simulink model "Grue_NL_corrNL"  (R2018b)
settings: Solver=ode1  StartTime=0.0  StopTime=dt  FixedStep=1e-2  RelTol=1e-3  EnableMultiTasking=on
values from neighbouring files (symbols this model uses):
  a = (Rini-zh)/(Dini-xh)^2    [Ini_Grue.m]
  b = 0.4    [Ini_Grue.m]
  C0 = m*g*b    (= 2000)    [Ini_Grue.m]
  Cd = 20    [Ini_Grue.m]
  coeff_phi = [6/Deltat^5 -15/Deltat^4 10/Deltat^3 0 0 0]    [Ini_Grue.m]
  coeff_phi2 = [-20/Deltat^7 70/Deltat^6 -84/Deltat^5 35/Deltat^4 0 0 0 0]    [Ini_Grue.m]
  Cr = 20    [Ini_Grue.m]    (also in plot_things.m = Cr*kc)
  Dfin = 20    [Ini_Grue.m]
  Dini = 0    [Ini_Grue.m]
  ed = omega0/100    [Ini_Grue.m]    (also in plot_things.m = omega0/e)
  er = ed    [Ini_Grue.m]    (also in plot_things.m = omega0/e)
  g = 10    [Ini_Grue.m]
  J = 50    [Ini_Grue.m]
  m = 500    [Ini_Grue.m]    (also in plot_things.m)
  Mc = 5000    [Ini_Grue.m]
  R = 15    [Ini_Grue.m]
  Rfin = 15    [Ini_Grue.m]
  Rini = 15    [Ini_Grue.m]
  xh = (Dini+sqrt((Rini-zh)/(Rfin-zh))*Dfin)/(1+sqrt((Rini-zh)/(Rfin-zh)))    [Ini_Grue.m]
  zh = 1    [Ini_Grue.m]
settings Model: Creator=abbasturki  LastModifiedBy=pac
settings DataIOCC: LimitDataPoints=on  SaveFormat=Array  SignalLoggingSaveFormat=ModelDataLogs
settings OptimizationCC: ExpressionDepthLimit=2147483647  LifeSpan=inf
settings DebuggingCC: UnderspecifiedInitializationDetection=Classic  MergeDetectMultiDrivingBlocksExec=none  SolverPrmCheckMsg=warning  FcnCallInpInsideContextMsg=warning  StateNameClashWarn=warning  SFUnexpectedBacktrackingDiag=warning  SFNoUnconditionalDefaultTransitionDiag=warning  SFExecutionAtInitializationDiag=none
settings HardwareCC: ProdBitPerPointer=32  ProdBitPerSizeT=32  ProdBitPerPtrDiffT=32  ProdLargestAtomicFloat=None  ProdIntDivRoundTo=Undefined  ProdEndianess=Unspecified  ProdWordSize=32  ProdHWDeviceType=32-bit Generic
settings ModelReferenceCC: PropagateSignalLabelsOutOfModel=off
settings SFSimCC: SimUseLocalCustomCode=off
settings RTWCC: RTWUseLocalCustomCode=off
settings CodeAppCC: StateflowObjectComments=on
settings GRTTargetCC: TargetLangStandard=C89/C90 (ANSI)  GeneratePreprocessorConditionals=Disable all  CombineOutputUpdateFcns=off  GRTInterface=on
settings ConfigComp: CovMetricSettings=dw  CovHtmlReporting=on  CovSaveCumulativeToWorkspaceVar=on  CovSaveSingleToWorkspaceVar=on  CovExternalEMLEnable=off

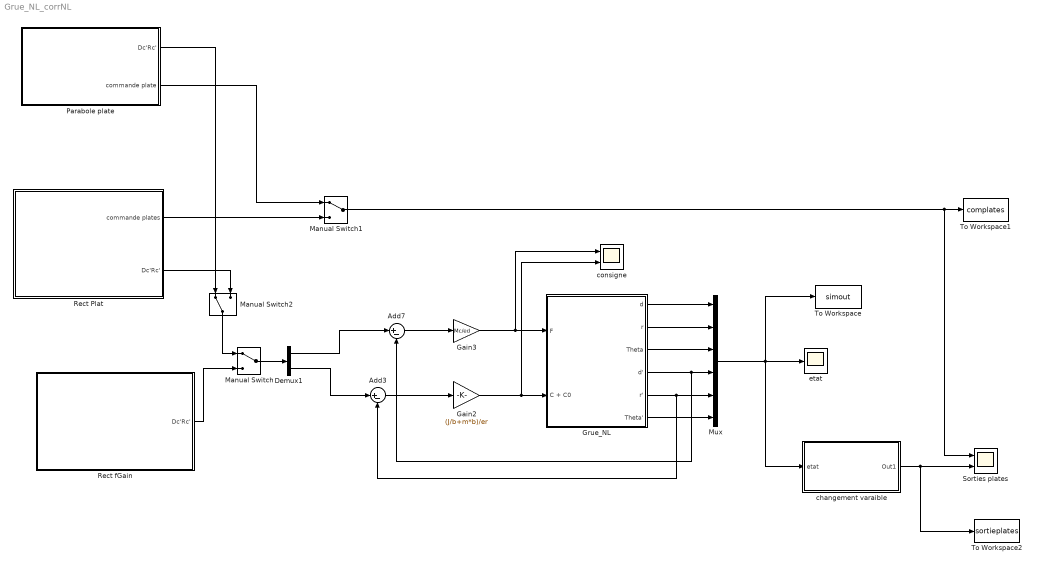
== system Grue_NL_corrNL ==
  Add3 : Sum  Inputs=|+-
  Add7 : Sum  Inputs=|+-
  Demux1 : Demux  Outputs=2
  Gain2 : Gain  Gain=(J/b+m*b)/er
  Gain3 : Gain  Gain=Mc/ed
  Grue_NL : Subsystem
  Manual Switch : ManualSwitch
  Manual Switch1 : ManualSwitch
  Manual Switch2 : ManualSwitch
  Mux : Mux  Inputs=6
  Parabole plate : Subsystem
  Rect Plat : Subsystem
  "Rect fGain " : Subsystem
  Sorties plates : Scope  NumInputPorts=2
  To Workspace : ToWorkspace  VariableName=simout  SaveFormat=Timeseries  SampleTime=-1
  To Workspace1 : ToWorkspace  VariableName=complates  SaveFormat=Timeseries  SampleTime=-1
  To Workspace2 : ToWorkspace  VariableName=sortieplates  SaveFormat=Timeseries  SampleTime=-1
  changement varaible : Subsystem
  consigne : Scope  NumInputPorts=2
  etat : Scope
  wires:
  Grue_NL/1(d) -> Mux/1
  Grue_NL/2(r) -> Mux/2
  Grue_NL/3(Theta) -> Mux/3
  Grue_NL/6(Theta') -> Mux/6
  Mux/1 -> changement varaible/1(etat), etat/1, To Workspace/1
  Gain3/1 -> consigne/1, Grue_NL/1(F)
  Gain2/1 -> consigne/2, Grue_NL/2(C + C0)
  Add7/1 -> Gain3/1
  Grue_NL/5(r') -> Add3/2, Mux/5
  Grue_NL/4(d') -> Add7/2, Mux/4
  Add3/1 -> Gain2/1
  Manual Switch/1 -> Demux1/1
  "Rect fGain "/1(Dc'Rc') -> Manual Switch/2
  Demux1/1 -> Add7/1
  Demux1/2 -> Add3/1
  changement varaible/1(Out1) -> To Workspace2/1, Sorties plates/2
  Parabole plate/2(commande plate) -> Manual Switch1/1
  Rect Plat/1(commande plates) -> Manual Switch1/2
  Manual Switch1/1 -> Sorties plates/1, To Workspace1/1
  Manual Switch2/1 -> Manual Switch/1
  Rect Plat/2(Dc'Rc') -> Manual Switch2/2
  Parabole plate/1(Dc'Rc') -> Manual Switch2/1

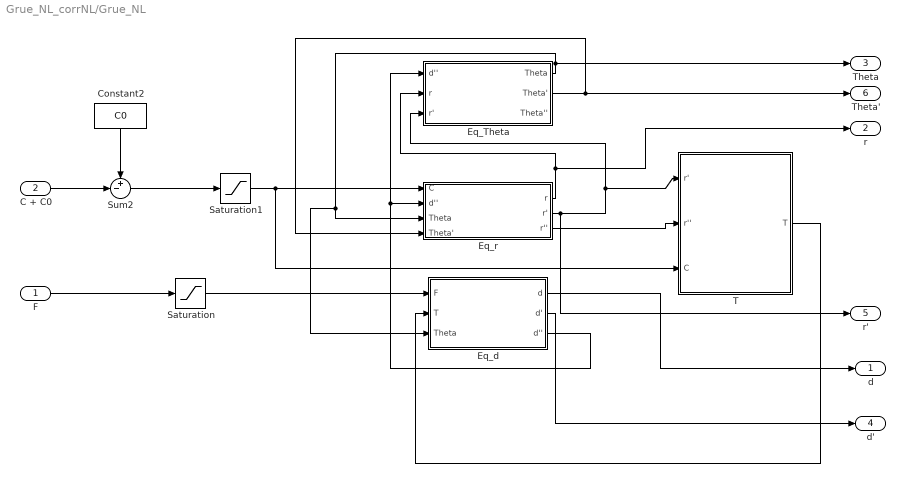
== system Grue_NL_corrNL/Grue_NL ==
  F : Inport
  C + C0 : Inport  Port=2
  Constant2 : Constant  Value=C0
  Eq_Theta : Subsystem
  Eq_d : Subsystem
  Eq_r : Subsystem
  Saturation : Saturate  UpperLimit=1e4  LowerLimit=-1e4
  Saturation1 : Saturate  UpperLimit=3e3  LowerLimit=-3e3
  Sum2 : Sum  Inputs=+-|
  T : Subsystem
  d : Outport
  r : Outport  Port=2
  Theta : Outport  Port=3
  d' : Outport  Port=4
  r' : Outport  Port=5
  Theta' : Outport  Port=6
  wires:
  Eq_r/2(r') -> Eq_Theta/3(r'), T/1(r'), r'/1
  Eq_r/1(r) -> Eq_Theta/2(r), r/1
  Eq_d/3(d'') -> Eq_Theta/1(d''), Eq_r/2(d'')
  Eq_d/2(d') -> d'/1
  Eq_Theta/1(Theta) -> Eq_d/3(Theta), Eq_r/3(Theta), Theta/1
  Eq_Theta/2(Theta') -> Eq_r/4(Theta'), Theta'/1
  Eq_r/3(r'') -> T/2(r'')
  F/1 -> Saturation/1
  T/1(T) -> Eq_d/2(T)
  Eq_d/1(d) -> d/1
  Saturation/1 -> Eq_d/1(F)
  Saturation1/1 -> Eq_r/1(C), T/3(C)
  Constant2/1 -> Sum2/1
  Sum2/1 -> Saturation1/1
  C + C0/1 -> Sum2/2

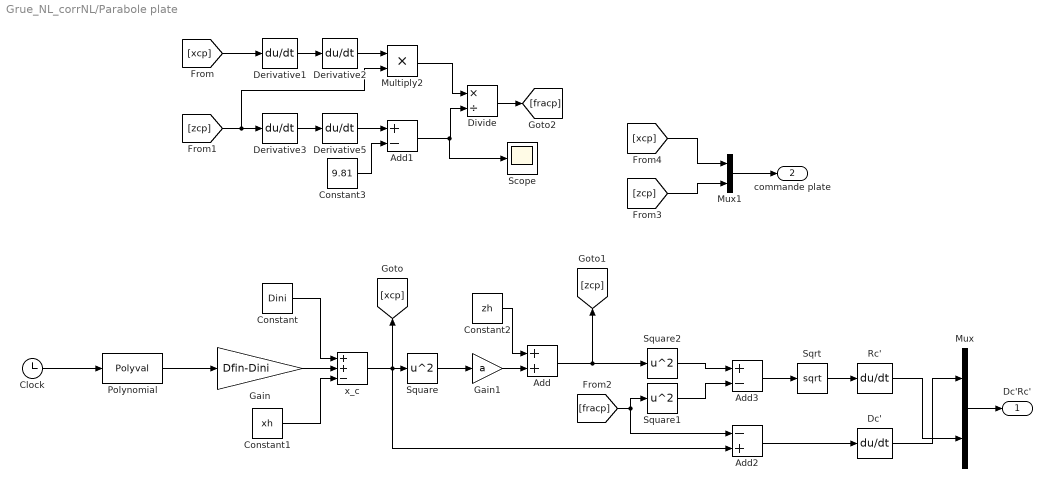
== system Grue_NL_corrNL/Parabole plate ==
  Add : Sum
  Add1 : Sum  Inputs=+-
  Add2 : Sum  Inputs=-+
  Add3 : Sum  Inputs=+-
  Clock : Clock
  Constant : Constant  Value=Dini
  Constant1 : Constant  Value=xh
  Constant2 : Constant  Value=zh
  Constant3 : Constant  Value=9.81
  Dc' : Derivative
  Derivative{1..3,5} (4 alike) : Derivative
  Divide : Product  Inputs=*/
  Gain : Gain  Gain=Dfin-Dini
  Gain1 : Gain  Gain=a
  Multiply2 : Product
  Mux : Mux  Inputs=2
  Mux1 : Mux  Inputs=2
  Polynomial : Polyval  Coefs=coeff_phi2
  Rc' : Derivative
  Scope : Scope
  Sqrt : Sqrt  SaturateOnIntegerOverflow=on
  Square : Math  Operator=square  SaturateOnIntegerOverflow=on
  Square1 : Math  Operator=square  SaturateOnIntegerOverflow=on
  Square2 : Math  Operator=square  SaturateOnIntegerOverflow=on
  x_c : Sum  Inputs=++-
  Dc'Rc' : Outport
  commande plate : Outport  Port=2
  wires:
  Constant/1 -> x_c/1
  Polynomial/1 -> Gain/1
  Square/1 -> Gain1/1
  Gain1/1 -> Add/2
  Gain/1 -> x_c/2
  Constant1/1 -> x_c/3
  Constant2/1 -> Add/1
  Clock/1 -> Polynomial/1
  Derivative2/1 -> Multiply2/1
  Divide/1 -> [fracp]
  Derivative3/1 -> Derivative5/1
  Derivative1/1 -> Derivative2/1
  [zcp] -> Multiply2/2, Derivative3/1
  Multiply2/1 -> Divide/1
  Add1/1 -> Scope/1, Divide/2
  Constant3/1 -> Add1/2
  Derivative5/1 -> Add1/1
  [xcp] -> Derivative1/1
  x_c/1 -> Add2/2, [xcp], Square/1
  [fracp] -> Add2/1, Square1/1
  Rc'/1 -> Mux/2
  Add2/1 -> Dc'/1
  Mux/1 -> Dc'Rc'/1
  Dc'/1 -> Mux/1
  Sqrt/1 -> Rc'/1
  Add/1 -> [zcp], Square2/1
  Square2/1 -> Add3/1
  Square1/1 -> Add3/2
  Add3/1 -> Sqrt/1
  Mux1/1 -> commande plate/1
  [xcp] -> Mux1/1
  [zcp] -> Mux1/2

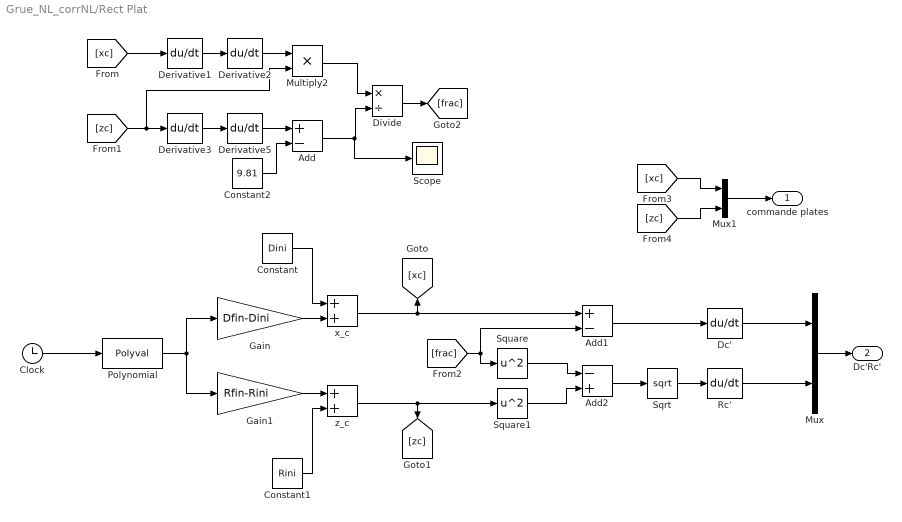
== system Grue_NL_corrNL/Rect Plat ==
  Add : Sum  Inputs=+-
  Add1 : Sum  Inputs=+-
  Add2 : Sum  Inputs=-+
  Clock : Clock
  Constant : Constant  Value=Dini
  Constant1 : Constant  Value=Rini
  Constant2 : Constant  Value=9.81
  Dc' : Derivative
  Derivative{1..3,5} (4 alike) : Derivative
  Divide : Product  Inputs=*/
  Gain : Gain  Gain=Dfin-Dini
  Gain1 : Gain  Gain=Rfin-Rini
  Multiply2 : Product
  Mux : Mux  Inputs=2
  Mux1 : Mux  Inputs=2
  Polynomial : Polyval  Coefs=coeff_phi2
  Rc' : Derivative
  Scope : Scope
  Sqrt : Sqrt  SaturateOnIntegerOverflow=on
  Square : Math  Operator=square  SaturateOnIntegerOverflow=on
  Square1 : Math  Operator=square  SaturateOnIntegerOverflow=on
  x_c : Sum
  z_c : Sum
  commande plates : Outport
  Dc'Rc' : Outport  Port=2
  wires:
  Gain1/1 -> z_c/1
  Square/1 -> Add2/1
  Derivative2/1 -> Multiply2/1
  Sqrt/1 -> Rc'/1
  Rc'/1 -> Mux/2
  Add2/1 -> Sqrt/1
  Add/1 -> Scope/1, Divide/2
  [zc] -> Multiply2/2, Derivative3/1
  Add1/1 -> Dc'/1
  z_c/1 -> Square1/1, [zc]
  Clock/1 -> Polynomial/1
  Polynomial/1 -> Gain/1, Gain1/1
  Multiply2/1 -> Divide/1
  Dc'/1 -> Mux/1
  Derivative3/1 -> Derivative5/1
  Derivative1/1 -> Derivative2/1
  Constant2/1 -> Add/2
  [xc] -> Derivative1/1
  Gain/1 -> x_c/2
  x_c/1 -> Add1/1, [xc]
  Constant1/1 -> z_c/2
  Constant/1 -> x_c/1
  Derivative5/1 -> Add/1
  Square1/1 -> Add2/2
  Divide/1 -> [frac]
  [frac] -> Add1/2, Square/1
  Mux/1 -> Dc'Rc'/1
  [xc] -> Mux1/1
  [zc] -> Mux1/2
  Mux1/1 -> commande plates/1

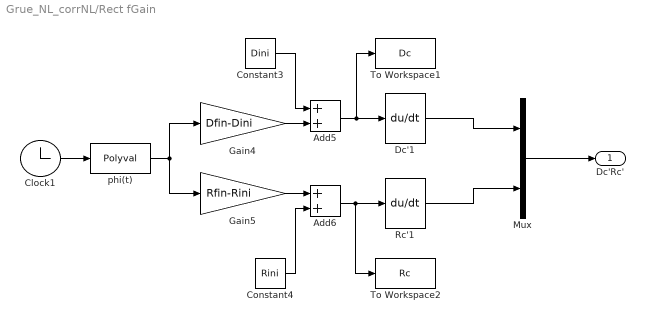
== system Grue_NL_corrNL/Rect fGain  ==
  Add5 : Sum
  Add6 : Sum
  Clock1 : Clock
  Constant3 : Constant  Value=Dini
  Constant4 : Constant  Value=Rini
  Dc'1 : Derivative
  Gain4 : Gain  Gain=Dfin-Dini
  Gain5 : Gain  Gain=Rfin-Rini
  Mux : Mux  Inputs=2
  Rc'1 : Derivative
  To Workspace1 : ToWorkspace  VariableName=Dc  SaveFormat=Timeseries  SampleTime=-1
  To Workspace2 : ToWorkspace  VariableName=Rc  SaveFormat=Timeseries  SampleTime=-1
  phi(t) : Polyval  Coefs=coeff_phi
  Dc'Rc' : Outport
  wires:
  Constant4/1 -> Add6/2
  Gain5/1 -> Add6/1
  Clock1/1 -> phi(t)/1
  Add5/1 -> To Workspace1/1, Dc'1/1
  Constant3/1 -> Add5/1
  Add6/1 -> To Workspace2/1, Rc'1/1
  phi(t)/1 -> Gain4/1, Gain5/1
  Gain4/1 -> Add5/2
  Rc'1/1 -> Mux/2
  Mux/1 -> Dc'Rc'/1
  Dc'1/1 -> Mux/1

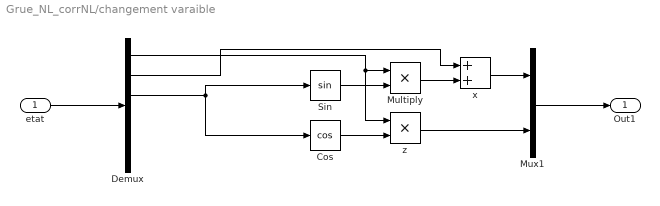
== system Grue_NL_corrNL/changement varaible ==
  etat : Inport
  Cos : Trigonometry  Operator=cos
  Demux : Demux  Outputs=6
  Multiply : Product
  Mux1 : Mux  Inputs=2
  Sin : Trigonometry
  x : Sum
  z : Product
  Out1 : Outport
  wires:
  Cos/1 -> z/2
  Multiply/1 -> x/2
  Sin/1 -> Multiply/2
  Demux/3 -> Cos/1, Sin/1
  z/1 -> Mux1/2
  Mux1/1 -> Out1/1
  etat/1 -> Demux/1
  Demux/1 -> z/1, Multiply/1
  x/1 -> Mux1/1
  Demux/2 -> x/1

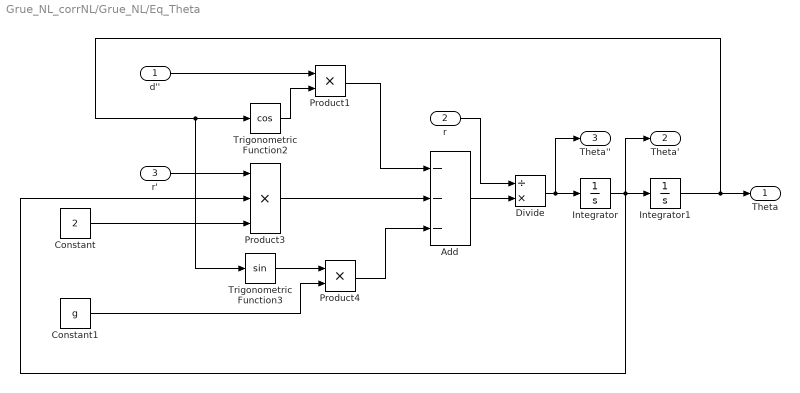
== system Grue_NL_corrNL/Grue_NL/Eq_Theta ==
  d'' : Inport
  r : Inport  Port=2
  r' : Inport  Port=3
  Add : Sum  Inputs=---
  Constant : Constant  Value=2
  Constant1 : Constant  Value=g
  Divide : Product  Inputs=/*
  Integrator : Integrator
  Integrator1 : Integrator
  Product1 : Product  RndMeth=Zero
  Product3 : Product  Inputs=3  RndMeth=Zero
  Product4 : Product  RndMeth=Zero
  Trigonometric Function2 : Trigonometry  Operator=cos
  Trigonometric Function3 : Trigonometry
  Theta : Outport
  Theta' : Outport  Port=2
  Theta'' : Outport  Port=3
  wires:
  d''/1 -> Product1/1
  Trigonometric Function2/1 -> Product1/2
  r'/1 -> Product3/1
  Constant/1 -> Product3/3
  Trigonometric Function3/1 -> Product4/1
  Constant1/1 -> Product4/2
  Product1/1 -> Add/1
  Product3/1 -> Add/2
  Product4/1 -> Add/3
  r/1 -> Divide/1
  Add/1 -> Divide/2
  Divide/1 -> Integrator/1, Theta''/1
  Integrator/1 -> Integrator1/1, Product3/2, Theta'/1
  Integrator1/1 -> Theta/1, Trigonometric Function2/1, Trigonometric Function3/1

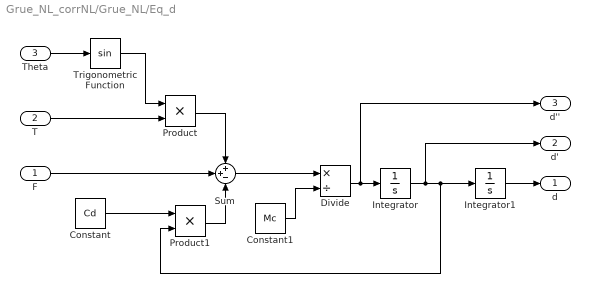
== system Grue_NL_corrNL/Grue_NL/Eq_d ==
  F : Inport
  T : Inport  Port=2
  Theta : Inport  Port=3
  Constant : Constant  Value=Cd
  Constant1 : Constant  Value=Mc
  Divide : Product  Inputs=*/
  Integrator : Integrator
  Integrator1 : Integrator
  Product : Product  RndMeth=Zero
  Product1 : Product  RndMeth=Zero
  Sum : Sum  Inputs=++-
  Trigonometric Function : Trigonometry
  d : Outport
  d' : Outport  Port=2
  d'' : Outport  Port=3
  wires:
  Product/1 -> Sum/1
  Trigonometric Function/1 -> Product/1
  Product1/1 -> Sum/3
  Constant/1 -> Product1/1
  Sum/1 -> Divide/1
  Constant1/1 -> Divide/2
  Divide/1 -> Integrator/1, d''/1
  Integrator/1 -> Integrator1/1, Product1/2, d'/1
  F/1 -> Sum/2
  T/1 -> Product/2
  Theta/1 -> Trigonometric Function/1
  Integrator1/1 -> d/1

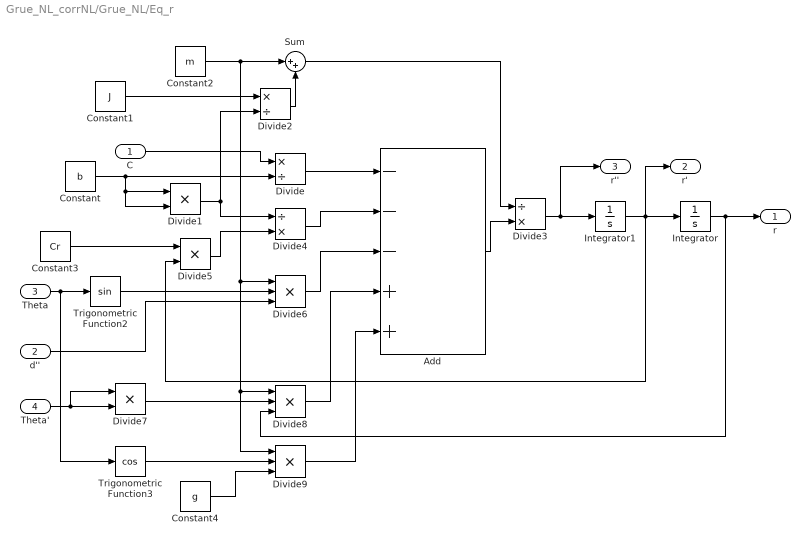
== system Grue_NL_corrNL/Grue_NL/Eq_r ==
  C : Inport
  d'' : Inport  Port=2
  Theta : Inport  Port=3
  Theta' : Inport  Port=4
  Add : Sum  Inputs=---++
  Constant : Constant  Value=b
  Constant1 : Constant  Value=J
  Constant2 : Constant  Value=m
  Constant3 : Constant  Value=Cr
  Constant4 : Constant  Value=g
  Divide : Product  Inputs=*/
  Divide1 : Product  Inputs=**
  Divide2 : Product  Inputs=*/
  Divide3 : Product  Inputs=/*
  Divide4 : Product  Inputs=/*
  Divide5 : Product  Inputs=**
  Divide6 : Product  Inputs=***
  Divide7 : Product  Inputs=**
  Divide8 : Product  Inputs=***
  Divide9 : Product  Inputs=***
  Integrator : Integrator  InitialCondition=R
  Integrator1 : Integrator
  Sum : Sum  Inputs=|++
  Trigonometric Function2 : Trigonometry
  Trigonometric Function3 : Trigonometry  Operator=cos
  r : Outport
  r' : Outport  Port=2
  r'' : Outport  Port=3
  wires:
  C/1 -> Divide/1
  Constant/1 -> Divide/2, Divide1/1, Divide1/2
  Divide/1 -> Add/1
  Constant2/1 -> Sum/1, Divide6/1, Divide8/1, Divide9/1
  Divide2/1 -> Sum/2
  Constant1/1 -> Divide2/1
  Divide1/1 -> Divide2/2, Divide4/1
  Sum/1 -> Divide3/1
  Add/1 -> Divide3/2
  Divide3/1 -> Integrator1/1, r''/1
  Integrator1/1 -> Integrator/1, Divide5/2, r'/1
  Constant3/1 -> Divide5/1
  Divide5/1 -> Divide4/2
  Divide4/1 -> Add/2
  Theta/1 -> Trigonometric Function2/1, Trigonometric Function3/1
  d''/1 -> Divide6/3
  Trigonometric Function2/1 -> Divide6/2
  Divide6/1 -> Add/3
  Theta'/1 -> Divide7/2, Divide7/1
  Divide7/1 -> Divide8/2
  Integrator/1 -> Divide8/3, r/1
  Divide8/1 -> Add/4
  Trigonometric Function3/1 -> Divide9/2
  Constant4/1 -> Divide9/3
  Divide9/1 -> Add/5

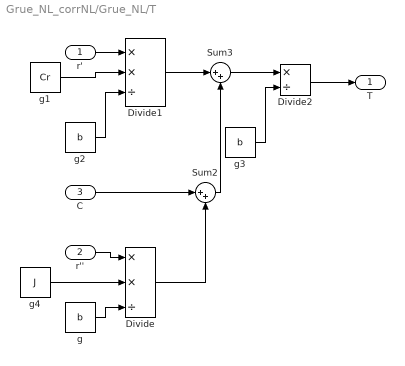
== system Grue_NL_corrNL/Grue_NL/T ==
  r' : Inport
  r'' : Inport  Port=2
  C : Inport  Port=3
  Divide : Product  Inputs=**/
  Divide1 : Product  Inputs=**/
  Divide2 : Product  Inputs=*/
  Sum2 : Sum  Inputs=|++
  Sum3 : Sum  Inputs=|++
  g : Constant  Value=b
  g1 : Constant  Value=Cr
  g2 : Constant  Value=b
  g3 : Constant  Value=b
  g4 : Constant  Value=J
  T : Outport
  wires:
  r''/1 -> Divide/1
  C/1 -> Sum2/1
  Divide/1 -> Sum2/2
  r'/1 -> Divide1/1
  g1/1 -> Divide1/2
  g2/1 -> Divide1/3
  Divide1/1 -> Sum3/1
  Sum2/1 -> Sum3/2
  Sum3/1 -> Divide2/1
  g3/1 -> Divide2/2
  Divide2/1 -> T/1
  g/1 -> Divide/3
  g4/1 -> Divide/2
